simulink model "DifferentialDriveControllerTemplate"  (R2021a)
settings: Solver=FixedStepAuto  StartTime=0.0  StopTime=inf  FixedStep=.1  RelTol=1e-3
libraries: robotlib x3
settings Model: EnablePacing=on  Creator=gavin  LastModifiedBy=gavin

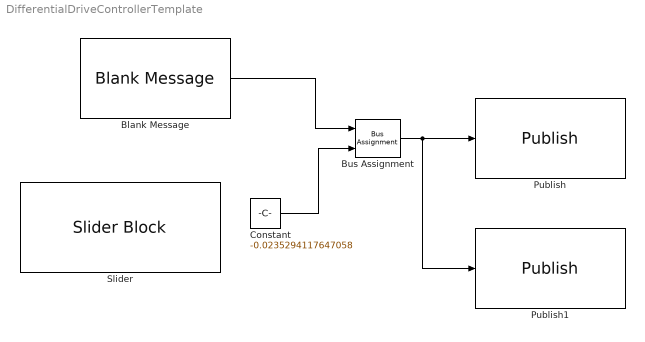
== system DifferentialDriveControllerTemplate ==
  Blank Message : robotlib/Blank Message  messageClass=Message  entityType=std_msgs/Float64  messageType=std_msgs/Float64  SampleTime=inf  legacyBusStruct=off
  Bus Assignment : BusAssignment  AssignedSignals=Data
  Constant : Constant  Value=-0.0235294117647058
  Publish : robotlib/Publish  topicSource=Select from ROS network  topic=/wheel_left_velocity_controller/command  messageType=std_msgs/Float64  legacyBusStruct=off  messageQueueLength=1
  Publish1 : robotlib/Publish  topicSource=Select from ROS network  topic=/wheel_right_velocity_controller/command  messageType=std_msgs/Float64  legacyBusStruct=off  messageQueueLength=1
  Slider : SliderBlock  ScaleMin=-2  ScaleMax=2
  wires:
  Blank Message/1 -> Bus Assignment/1
  Constant/1 -> Bus Assignment/2
  Bus Assignment/1 -> Publish1/1, Publish/1
